simulink model "Bitchplzwork"  (Simulink 9.3)
settings: Solver=VariableStepAuto  StartTime=0.0  StopTime=1  FixedStep=0.1
values from neighbouring files (symbols this model uses):
  C = 13.5e-4    (= 0.00135)    [inverter.m]
  L = 27e-3    (= 0.027)    [inverter.m]
  R = 0.001    [inverter.m]
  Tss = 2.5e-6    (= 2.5e-06)    [inverter.m]
undefined symbols (not defined in the file or in its folder): Acid, Hydride, Lead, Metal, Nickel
libraries: powerlib x39, powerlib_extras x9, simulink x6, powerlib_meascontrol x4, electricdrivelib x2, re_lib x2, dsparch4 x1
(part 2 of 2)

== system Bitchplzwork/Battery DC-DC converter /Battery Converter  Control/Subsystem4 ==
  S1 : Inport
  To Workspace1 : ToWorkspace  VariableName=S1  SampleTime=-1
  Zero-Order Hold : ZeroOrderHold  SampleTime=Tss
  wires:
  S1/1 -> Zero-Order Hold/1
  Zero-Order Hold/1 -> To Workspace1/1

== system Bitchplzwork/Battery DC-DC converter /Battery Converter  Control/Subsystem5 ==
  S2 : Inport
  To Workspace1 : ToWorkspace  VariableName=S2  SampleTime=-1
  Zero-Order Hold : ZeroOrderHold  SampleTime=Tss
  wires:
  S2/1 -> Zero-Order Hold/1
  Zero-Order Hold/1 -> To Workspace1/1

== system Bitchplzwork/Battery DC-DC converter /Battery Converter  Control/Subsystem6 ==
  Sign : Inport
  To Workspace1 : ToWorkspace  VariableName=Sign  SampleTime=-1
  Zero-Order Hold : ZeroOrderHold  SampleTime=Tss
  tag scope: Sign=global
  wires:
  Sign/1 -> Zero-Order Hold/1
  Zero-Order Hold/1 -> [Sign], To Workspace1/1

== system Bitchplzwork/Inverter Control/Iabc  - idq/abc  - alfa/beta ==
  abc : Inport
  Mux : Mux  Inputs=2
  d_s : Fcn  Expr=(-1/sqrt(3)*u(2))+(1/sqrt(3)*u(3))
  q_s : Fcn  Expr=(2/3)*u(1)-(1/3)*u(2)-(1/3)*u(3)
  alfa/beta : Outport
  wires:
  abc/1 -> q_s/1, d_s/1
  d_s/1 -> Mux/1
  q_s/1 -> Mux/2
  Mux/1 -> alfa/beta/1

== system Bitchplzwork/Inverter Control/Iabc  - idq/alfa/beta - dq ==
  alfa/beta : Inport
  theta : Inport  Port=2
  Mux : Mux  Inputs=2
  Mux1 : Mux  Inputs=2
  d : Fcn  Expr=u(2)*sin(u(3)) + u(1)*cos(u(3))
  q : Fcn  Expr=-u(1)*sin(u(3)) + u(2)*cos(u(3))
  d/q : Outport
  wires:
  d/1 -> Mux/1
  q/1 -> Mux/2
  Mux/1 -> d/q/1
  alfa/beta/1 -> Mux1/1
  theta/1 -> Mux1/2
  Mux1/1 -> d/1, q/1

== system Bitchplzwork/Inverter Control/Vabc  - vdq/abc  - alfa/beta ==
  abc : Inport
  Mux : Mux  Inputs=2
  d_s : Fcn  Expr=(-1/sqrt(3)*u(2))+(1/sqrt(3)*u(3))
  q_s : Fcn  Expr=(2/3)*u(1)-(1/3)*u(2)-(1/3)*u(3)
  alfa/beta : Outport
  wires:
  Mux/1 -> alfa/beta/1
  q_s/1 -> Mux/2
  d_s/1 -> Mux/1
  abc/1 -> d_s/1, q_s/1

== system Bitchplzwork/Inverter Control/Vabc  - vdq/alfa/beta - dq ==
  alfa/beta : Inport
  theta : Inport  Port=2
  Mux : Mux  Inputs=2
  Mux1 : Mux  Inputs=2
  d : Fcn  Expr=u(2)*sin(u(3)) + u(1)*cos(u(3))
  q : Fcn  Expr=-u(1)*sin(u(3)) + u(2)*cos(u(3))
  d/q : Outport
  wires:
  Mux1/1 -> q/1, d/1
  theta/1 -> Mux1/2
  alfa/beta/1 -> Mux1/1
  Mux/1 -> d/q/1
  q/1 -> Mux/2
  d/1 -> Mux/1

== system Bitchplzwork/Inverter Control/Vabc*  - vdq*/abc  - alfa/beta ==
  abc : Inport
  Mux : Mux  Inputs=2
  d_s : Fcn  Expr=(-1/sqrt(3)*u(2))+(1/sqrt(3)*u(3))
  q_s : Fcn  Expr=(2/3)*u(1)-(1/3)*u(2)-(1/3)*u(3)
  alfa/beta : Outport
  wires:
  abc/1 -> q_s/1, d_s/1
  d_s/1 -> Mux/1
  q_s/1 -> Mux/2
  Mux/1 -> alfa/beta/1

== system Bitchplzwork/Inverter Control/Vabc*  - vdq*/alfa/beta - dq ==
  alfa/beta : Inport
  theta : Inport  Port=2
  Mux : Mux  Inputs=2
  Mux1 : Mux  Inputs=2
  d : Fcn  Expr=u(2)*sin(u(3)) + u(1)*cos(u(3))
  q : Fcn  Expr=-u(1)*sin(u(3)) + u(2)*cos(u(3))
  d/q : Outport
  wires:
  d/1 -> Mux/1
  q/1 -> Mux/2
  Mux/1 -> d/q/1
  alfa/beta/1 -> Mux1/1
  theta/1 -> Mux1/2
  Mux1/1 -> d/1, q/1

== system Bitchplzwork/Inverter Control/vdq - Vabc/alfa/beta - abc ==
  alfa/beta : Inport
  Mux : Mux  Inputs=3
  a : Fcn  Expr=u[2]
  b : Fcn  Expr=-sqrt(3)/2*u[1]-0.5*u[2]
  c : Fcn  Expr=sqrt(3)/2*u[1]-0.5*u[2]
  abc : Outport
  tag scope: Vca_ref=global, Vcb_ref=global, Vcc_ref=global
  wires:
  alfa/beta/1 -> c/1, a/1, b/1
  Mux/1 -> abc/1
  c/1 -> Mux/3, [Vcc_ref]
  b/1 -> Mux/2, [Vcb_ref]
  a/1 -> Mux/1, [Vca_ref]

== system Bitchplzwork/Inverter Control/vdq - Vabc/d/q - alfa/beta ==
  d/q : Inport
  tita : Inport  Port=2
  Mux : Mux  Inputs=2
  Mux1 : Mux  Inputs=2
  a : Fcn  Expr=-u[2]*sin(u[3]) + u[1]*cos(u[3])
  b : Fcn  Expr=u[1]*sin(u[3]) + u[2]*cos(u[3])
  alfa/beta : Outport
  wires:
  Mux1/1 -> b/1, a/1
  tita/1 -> Mux1/2
  d/q/1 -> Mux1/1
  a/1 -> Mux/1
  b/1 -> Mux/2
  Mux/1 -> alfa/beta/1

== matlab function PV array 1/MPPT ==
  settings: updateMethod=DISCRETE
  data: vpv input double; duty output double; ipv input double; delta input double
function duty  = MPPT_algorithm(vpv,ipv,delta)

duty_init = 0.1;
duty_min = 0;
duty_max = 0.85;


persistent Vold Pold duty_old;


if isempty(Vold)
    Vold=0;
    Pold=0;
    duty_old=duty_init;
end
P=vpv*ipv;
dV= vpv - Vold;
dP= P - Pold;

if dP == 0 && vpv>30
    if dP < 0 
        if dV < 0 
            duty = duty_old - delta ;
        else 
            duty = duty_old + delta ;
        end 
    else 
        if dV < 0 
            duty = duty_old + delta;
        else 
            duty = duty_old - delta;
        end 
    end 
else 
    duty = duty_old;
end 
if duty >= duty_max
    duty=duty_max;
elseif duty<duty_min
    duty=duty_min;
end 

duty_old=duty;
Vold=vpv;
Pold=P;

== matlab function Subsystem/MATLAB Function ==
  data: SOC input double; LoadOn output double; ChargingOn output double
function[LoadOn,ChargingOn] = fcn(SOC)
%#codegen
       LoadOn=1;
       ChargingOn=0;
if     (SOC>=80)
       LoadOn=1;
       ChargingOn=0;
end

if    (SOC<40)
      LoadOn=0;
      ChargingOn=1;
end

== matlab function Battery DC-DC converter /MATLAB Function ==
  data: SOC input double; LoadOn output double; ChargingOn output double
function[LoadOn,ChargingOn] = fcn(SOC)
%#codegen
       LoadOn=1;
       ChargingOn=0;
if     (SOC>=80)
       LoadOn=1;
       ChargingOn=0;
end

if    (SOC<40)
      LoadOn=0;
      ChargingOn=1;
end
